simulink model "zero_to_hero_sect7to8"  (R2023a)
settings: Solver=VariableStepAuto  StartTime=0.0  StopTime=runtime  RelTol=1e-3
values from neighbouring files (symbols this model uses):
  b = 50    [zero_to_hero_sect10_script.m]    (also in zero_to_hero_sect1to5_script.m = 0.1; zero_to_hero_sect7to8_script.m = 10)
  D_Control = 1    [zero_to_hero_sect7to8_script.m]
  I_Control = 1    [zero_to_hero_sect7to8_script.m]
  k = 0.3    [zero_to_hero_sect1to5_script.m]    (also in zero_to_hero_sect7to8_script.m = 20)
  K_D = 50    [zero_to_hero_sect7to8_script.m]
  K_I = 300    [zero_to_hero_sect7to8_script.m]
  K_P = 350    [zero_to_hero_sect7to8_script.m]
  m = 1000    [zero_to_hero_sect10_script.m]    (also in zero_to_hero_sect1to5_script.m = 1; zero_to_hero_sect7to8_script.m = 1)
  P_Control = 1    [zero_to_hero_sect7to8_script.m]
  step_val = 1    [zero_to_hero_sect7to8_script.m]
settings Model: Creator=fycce  LastModifiedBy=fycce
settings DataIOCC: SaveOutput=off  SaveTime=off  ReturnWorkspaceOutputs=off

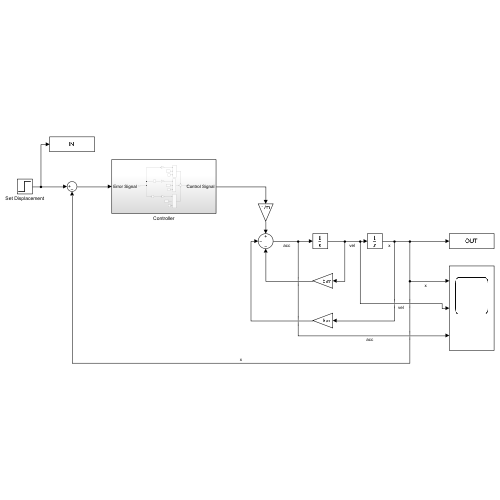
[thumbnail: Simulink's stored preview of the top-level diagram]
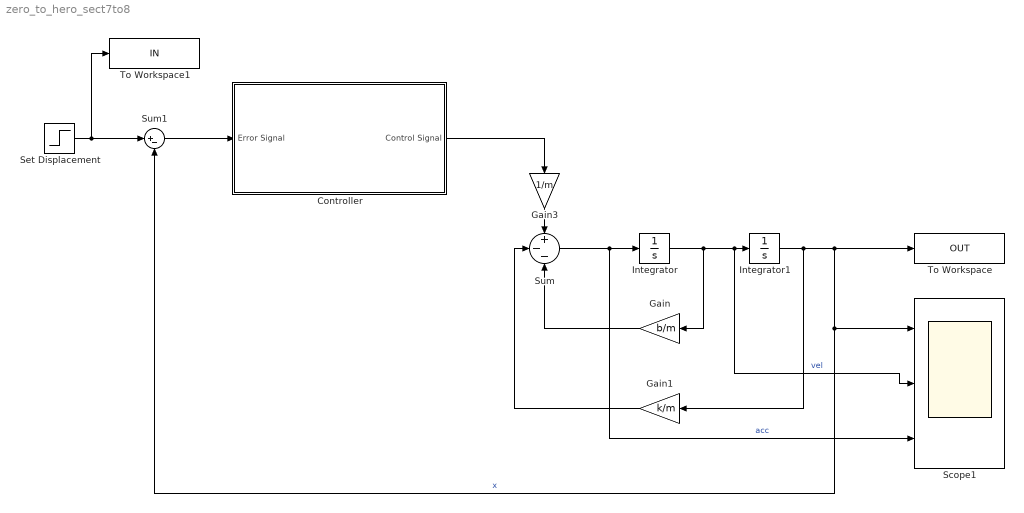
== system zero_to_hero_sect7to8 ==
  Controller : Subsystem
  Gain : Gain  Gain=b/m
  Gain1 : Gain  Gain=k/m
  Gain3 : Gain  Gain=1/m
  Integrator : Integrator
  Integrator1 : Integrator
  Scope1 : Scope  NumInputPorts=3
  Set Displacement : Step  After=step_val  SampleTime=0
  Sum : Sum  Inputs=+--
  Sum1 : Sum  Inputs=|+-
  To Workspace : ToWorkspace  VariableName=OUT  SaveFormat=Timeseries  SampleTime=-1
  To Workspace1 : ToWorkspace  VariableName=IN  SaveFormat=Timeseries  SampleTime=-1
  wires:
  Gain1/1 -> Sum/2
  Gain/1 -> Sum/3
  Integrator1/1 -> Sum1/2, Scope1/1, To Workspace/1, Gain1/1  "x"
  Sum/1 -> Scope1/3, Integrator/1  "acc"
  Integrator/1 -> Gain/1, Scope1/2, Integrator1/1  "vel"
  Gain3/1 -> Sum/1
  Controller/1(Control Signal) -> Gain3/1
  Set Displacement/1 -> To Workspace1/1, Sum1/1
  Sum1/1 -> Controller/1(Error Signal)

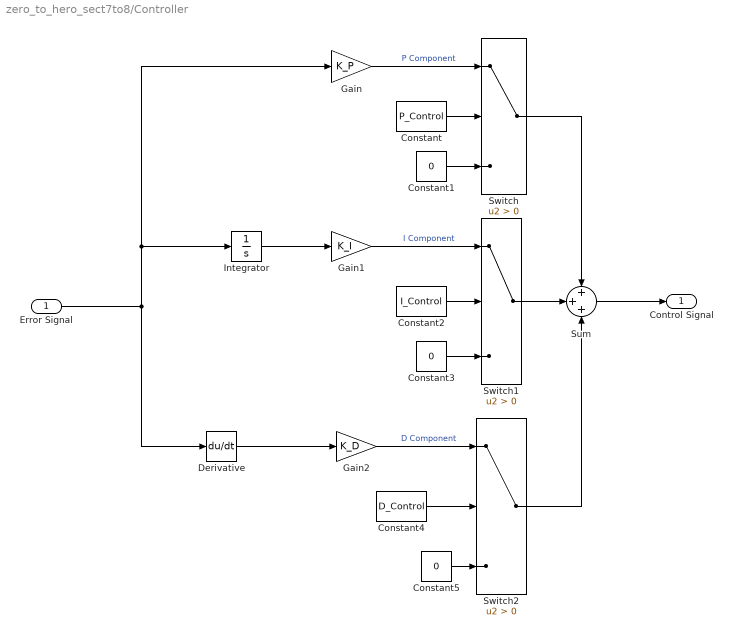
== system zero_to_hero_sect7to8/Controller ==
  Error Signal : Inport
  Constant : Constant  Value=P_Control
  Constant1 : Constant  Value=0
  Constant2 : Constant  Value=I_Control
  Constant3 : Constant  Value=0
  Constant4 : Constant  Value=D_Control
  Constant5 : Constant  Value=0
  Derivative : Derivative
  Gain : Gain  Gain=K_P
  Gain1 : Gain  Gain=K_I
  Gain2 : Gain  Gain=K_D
  Integrator : Integrator
  Sum : Sum  Inputs=+++
  Switch : Switch  Criteria=u2 > Threshold  SaturateOnIntegerOverflow=off  InputSameDT=off
  Switch1 : Switch  Criteria=u2 > Threshold  SaturateOnIntegerOverflow=off  InputSameDT=off
  Switch2 : Switch  Criteria=u2 > Threshold  SaturateOnIntegerOverflow=off  InputSameDT=off
  Control Signal : Outport
  wires:
  Gain2/1 -> Switch2/1  "D Component"
  Sum/1 -> Control Signal/1
  Derivative/1 -> Gain2/1
  Error Signal/1 -> Gain/1, Integrator/1, Derivative/1
  Gain/1 -> Switch/1  "P Component"
  Integrator/1 -> Gain1/1
  Switch/1 -> Sum/1
  Constant/1 -> Switch/2
  Constant1/1 -> Switch/3
  Constant3/1 -> Switch1/3
  Constant2/1 -> Switch1/2
  Constant5/1 -> Switch2/3
  Constant4/1 -> Switch2/2
  Gain1/1 -> Switch1/1  "I Component"
  Switch1/1 -> Sum/2
  Switch2/1 -> Sum/3
